simulink model "matrixCreator"  (R2017b)
settings: Solver=VariableStepAuto  StartTime=0.0  StopTime=10.0  RelTol=1e-3
undefined symbols (not defined in the file or in its folder): A
settings Model: Creator=rablanco.ext  LastModifiedBy=rablanco.ext

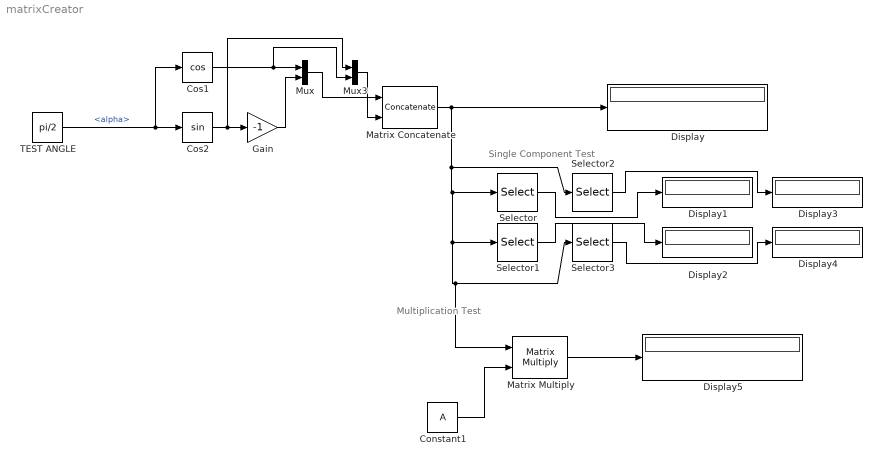
== system matrixCreator ==
  note: Single Component Test
  note: Multiplication Test
  Constant1 : Constant  Value=A
  Cos1 : Trigonometry  Operator=cos  OutputSignalType=real
  Cos2 : Trigonometry  OutputSignalType=real
  Display{,1..5} (6 alike) : Display
  Gain : Gain  Gain=-1
  Matrix Concatenate : Concatenate  Mode=Multidimensional array  ConcatenateDimension=2
  Matrix Multiply : Product  Multiplication=Matrix(*)
  Mux : Mux  Inputs=2
  Mux3 : Mux  Inputs=2
  Selector : Selector  NumberOfDimensions=2  InputPortWidth=3  IndexOptions=Index vector (dialog),Index vector (dialog)  Indices=1,1  OutputSizes=1,1
  Selector1 : Selector  NumberOfDimensions=2  InputPortWidth=3  IndexOptions=Index vector (dialog),Index vector (dialog)  Indices=2,1  OutputSizes=1,1
  Selector2 : Selector  NumberOfDimensions=2  InputPortWidth=3  IndexOptions=Index vector (dialog),Index vector (dialog)  Indices=1,2  OutputSizes=1,1
  Selector3 : Selector  NumberOfDimensions=2  InputPortWidth=3  IndexOptions=Index vector (dialog),Index vector (dialog)  Indices=2,2  OutputSizes=1,1
  TEST ANGLE : Constant  Value=pi/2
  wires:
  Cos1/1 -> Mux3/2, Mux/1
  Matrix Concatenate/1 -> Selector2/1, Selector1/1, Matrix Multiply/1, Selector3/1, Selector/1, Display/1
  Mux3/1 -> Matrix Concatenate/2
  TEST ANGLE/1 -> Cos1/1, Cos2/1  "<alpha>"
  Gain/1 -> Mux/2
  Cos2/1 -> Mux3/1, Gain/1
  Mux/1 -> Matrix Concatenate/1
  Selector/1 -> Display1/1
  Selector2/1 -> Display3/1
  Selector3/1 -> Display4/1
  Selector1/1 -> Display2/1
  Constant1/1 -> Matrix Multiply/2
  Matrix Multiply/1 -> Display5/1
